simulink model "gm_DUALportRAMinterface_v3_vnl"  (R2024a)
settings: Solver=FixedStepDiscrete  StartTime=0.0  StopTime=20  RelTol=1e-3
undefined symbols (not defined in the file or in its folder): magnitude, Ts
libraries: hdlsllib x419, hdlmdlgenlib x103, embmathops x12, simulink x5, dsphdlxfrm2 x2
(part 11 of 11)

== system gm_DUALportRAMinterface_v3_vnl/PL_vnl/integration_block1/GA_main/coefficent_array1/individual1/Subsystem6 ==
  reg_in : Inport
  enable : Inport  Port=2
  Delay : Delay  DelayLength=1  InitialCondition=0  SampleTime=Ts
  Switch : Switch  Criteria=u2 > Threshold  SaturateOnIntegerOverflow=off  InputSameDT=off
  reg_out : Outport
  wires:
  reg_in/1 -> Switch/1
  enable/1 -> Switch/2
  Switch/1 -> Delay/1
  Delay/1 -> Switch/3, reg_out/1

== system gm_DUALportRAMinterface_v3_vnl/PL_vnl/integration_block1/GA_main/coefficent_array1/individual2/Subsystem ==
  reg_in : Inport
  enable : Inport  Port=2
  Delay : Delay  DelayLength=1  InitialCondition=0  SampleTime=Ts
  Switch : Switch  Criteria=u2 > Threshold  SaturateOnIntegerOverflow=off  InputSameDT=off
  reg_out : Outport
  wires:
  reg_in/1 -> Switch/1
  enable/1 -> Switch/2
  Switch/1 -> Delay/1
  Delay/1 -> Switch/3, reg_out/1

== system gm_DUALportRAMinterface_v3_vnl/PL_vnl/integration_block1/GA_main/coefficent_array1/individual2/Subsystem1 ==
  reg_in : Inport
  enable : Inport  Port=2
  Delay : Delay  DelayLength=1  InitialCondition=0  SampleTime=Ts
  Switch : Switch  Criteria=u2 > Threshold  SaturateOnIntegerOverflow=off  InputSameDT=off
  reg_out : Outport
  wires:
  reg_in/1 -> Switch/1
  enable/1 -> Switch/2
  Switch/1 -> Delay/1
  Delay/1 -> Switch/3, reg_out/1

== system gm_DUALportRAMinterface_v3_vnl/PL_vnl/integration_block1/GA_main/coefficent_array1/individual2/Subsystem2 ==
  reg_in : Inport
  enable : Inport  Port=2
  Delay : Delay  DelayLength=1  InitialCondition=0  SampleTime=Ts
  Switch : Switch  Criteria=u2 > Threshold  SaturateOnIntegerOverflow=off  InputSameDT=off
  reg_out : Outport
  wires:
  reg_in/1 -> Switch/1
  enable/1 -> Switch/2
  Switch/1 -> Delay/1
  Delay/1 -> Switch/3, reg_out/1

== system gm_DUALportRAMinterface_v3_vnl/PL_vnl/integration_block1/GA_main/coefficent_array1/individual2/Subsystem3 ==
  reg_in : Inport
  enable : Inport  Port=2
  Delay : Delay  DelayLength=1  InitialCondition=0  SampleTime=Ts
  Switch : Switch  Criteria=u2 > Threshold  SaturateOnIntegerOverflow=off  InputSameDT=off
  reg_out : Outport
  wires:
  reg_in/1 -> Switch/1
  enable/1 -> Switch/2
  Switch/1 -> Delay/1
  Delay/1 -> Switch/3, reg_out/1

== system gm_DUALportRAMinterface_v3_vnl/PL_vnl/integration_block1/GA_main/coefficent_array1/individual2/Subsystem4 ==
  reg_in : Inport
  enable : Inport  Port=2
  Delay : Delay  DelayLength=1  InitialCondition=0  SampleTime=Ts
  Switch : Switch  Criteria=u2 > Threshold  SaturateOnIntegerOverflow=off  InputSameDT=off
  reg_out : Outport
  wires:
  reg_in/1 -> Switch/1
  enable/1 -> Switch/2
  Switch/1 -> Delay/1
  Delay/1 -> Switch/3, reg_out/1

== system gm_DUALportRAMinterface_v3_vnl/PL_vnl/integration_block1/GA_main/coefficent_array1/individual2/Subsystem5 ==
  reg_in : Inport
  enable : Inport  Port=2
  Delay : Delay  DelayLength=1  InitialCondition=0  SampleTime=Ts
  Switch : Switch  Criteria=u2 > Threshold  SaturateOnIntegerOverflow=off  InputSameDT=off
  reg_out : Outport
  wires:
  reg_in/1 -> Switch/1
  enable/1 -> Switch/2
  Switch/1 -> Delay/1
  Delay/1 -> Switch/3, reg_out/1

== system gm_DUALportRAMinterface_v3_vnl/PL_vnl/integration_block1/GA_main/coefficent_array1/individual2/Subsystem6 ==
  reg_in : Inport
  enable : Inport  Port=2
  Delay : Delay  DelayLength=1  InitialCondition=0  SampleTime=Ts
  Switch : Switch  Criteria=u2 > Threshold  SaturateOnIntegerOverflow=off  InputSameDT=off
  reg_out : Outport
  wires:
  Delay/1 -> reg_out/1, Switch/3
  Switch/1 -> Delay/1
  enable/1 -> Switch/2
  reg_in/1 -> Switch/1

== system gm_DUALportRAMinterface_v3_vnl/PL_vnl/integration_block1/GA_main/coefficent_array1/individual3/Subsystem ==
  reg_in : Inport
  enable : Inport  Port=2
  Delay : Delay  DelayLength=1  InitialCondition=0  SampleTime=Ts
  Switch : Switch  Criteria=u2 > Threshold  SaturateOnIntegerOverflow=off  InputSameDT=off
  reg_out : Outport
  wires:
  Delay/1 -> reg_out/1, Switch/3
  Switch/1 -> Delay/1
  enable/1 -> Switch/2
  reg_in/1 -> Switch/1

== system gm_DUALportRAMinterface_v3_vnl/PL_vnl/integration_block1/GA_main/coefficent_array1/individual3/Subsystem1 ==
  reg_in : Inport
  enable : Inport  Port=2
  Delay : Delay  DelayLength=1  InitialCondition=0  SampleTime=Ts
  Switch : Switch  Criteria=u2 > Threshold  SaturateOnIntegerOverflow=off  InputSameDT=off
  reg_out : Outport
  wires:
  Delay/1 -> reg_out/1, Switch/3
  Switch/1 -> Delay/1
  enable/1 -> Switch/2
  reg_in/1 -> Switch/1

== system gm_DUALportRAMinterface_v3_vnl/PL_vnl/integration_block1/GA_main/coefficent_array1/individual3/Subsystem2 ==
  reg_in : Inport
  enable : Inport  Port=2
  Delay : Delay  DelayLength=1  InitialCondition=0  SampleTime=Ts
  Switch : Switch  Criteria=u2 > Threshold  SaturateOnIntegerOverflow=off  InputSameDT=off
  reg_out : Outport
  wires:
  Delay/1 -> reg_out/1, Switch/3
  Switch/1 -> Delay/1
  enable/1 -> Switch/2
  reg_in/1 -> Switch/1

== system gm_DUALportRAMinterface_v3_vnl/PL_vnl/integration_block1/GA_main/coefficent_array1/individual3/Subsystem3 ==
  reg_in : Inport
  enable : Inport  Port=2
  Delay : Delay  DelayLength=1  InitialCondition=0  SampleTime=Ts
  Switch : Switch  Criteria=u2 > Threshold  SaturateOnIntegerOverflow=off  InputSameDT=off
  reg_out : Outport
  wires:
  Delay/1 -> reg_out/1, Switch/3
  Switch/1 -> Delay/1
  enable/1 -> Switch/2
  reg_in/1 -> Switch/1

== system gm_DUALportRAMinterface_v3_vnl/PL_vnl/integration_block1/GA_main/coefficent_array1/individual3/Subsystem4 ==
  reg_in : Inport
  enable : Inport  Port=2
  Delay : Delay  DelayLength=1  InitialCondition=0  SampleTime=Ts
  Switch : Switch  Criteria=u2 > Threshold  SaturateOnIntegerOverflow=off  InputSameDT=off
  reg_out : Outport
  wires:
  Delay/1 -> reg_out/1, Switch/3
  Switch/1 -> Delay/1
  enable/1 -> Switch/2
  reg_in/1 -> Switch/1

== system gm_DUALportRAMinterface_v3_vnl/PL_vnl/integration_block1/GA_main/coefficent_array1/individual3/Subsystem5 ==
  reg_in : Inport
  enable : Inport  Port=2
  Delay : Delay  DelayLength=1  InitialCondition=0  SampleTime=Ts
  Switch : Switch  Criteria=u2 > Threshold  SaturateOnIntegerOverflow=off  InputSameDT=off
  reg_out : Outport
  wires:
  Delay/1 -> reg_out/1, Switch/3
  Switch/1 -> Delay/1
  enable/1 -> Switch/2
  reg_in/1 -> Switch/1

== system gm_DUALportRAMinterface_v3_vnl/PL_vnl/integration_block1/GA_main/coefficent_array1/individual3/Subsystem6 ==
  reg_in : Inport
  enable : Inport  Port=2
  Delay : Delay  DelayLength=1  InitialCondition=0  SampleTime=Ts
  Switch : Switch  Criteria=u2 > Threshold  SaturateOnIntegerOverflow=off  InputSameDT=off
  reg_out : Outport
  wires:
  reg_in/1 -> Switch/1
  enable/1 -> Switch/2
  Switch/1 -> Delay/1
  Delay/1 -> Switch/3, reg_out/1

== system gm_DUALportRAMinterface_v3_vnl/PL_vnl/integration_block1/GA_main/coefficent_array1/individual4/Subsystem ==
  reg_in : Inport
  enable : Inport  Port=2
  Delay : Delay  DelayLength=1  InitialCondition=0  SampleTime=Ts
  Switch : Switch  Criteria=u2 > Threshold  SaturateOnIntegerOverflow=off  InputSameDT=off
  reg_out : Outport
  wires:
  reg_in/1 -> Switch/1
  enable/1 -> Switch/2
  Switch/1 -> Delay/1
  Delay/1 -> Switch/3, reg_out/1

== system gm_DUALportRAMinterface_v3_vnl/PL_vnl/integration_block1/GA_main/coefficent_array1/individual4/Subsystem1 ==
  reg_in : Inport
  enable : Inport  Port=2
  Delay : Delay  DelayLength=1  InitialCondition=0  SampleTime=Ts
  Switch : Switch  Criteria=u2 > Threshold  SaturateOnIntegerOverflow=off  InputSameDT=off
  reg_out : Outport
  wires:
  reg_in/1 -> Switch/1
  enable/1 -> Switch/2
  Switch/1 -> Delay/1
  Delay/1 -> Switch/3, reg_out/1

== system gm_DUALportRAMinterface_v3_vnl/PL_vnl/integration_block1/GA_main/coefficent_array1/individual4/Subsystem2 ==
  reg_in : Inport
  enable : Inport  Port=2
  Delay : Delay  DelayLength=1  InitialCondition=0  SampleTime=Ts
  Switch : Switch  Criteria=u2 > Threshold  SaturateOnIntegerOverflow=off  InputSameDT=off
  reg_out : Outport
  wires:
  reg_in/1 -> Switch/1
  enable/1 -> Switch/2
  Switch/1 -> Delay/1
  Delay/1 -> Switch/3, reg_out/1

== system gm_DUALportRAMinterface_v3_vnl/PL_vnl/integration_block1/GA_main/coefficent_array1/individual4/Subsystem3 ==
  reg_in : Inport
  enable : Inport  Port=2
  Delay : Delay  DelayLength=1  InitialCondition=0  SampleTime=Ts
  Switch : Switch  Criteria=u2 > Threshold  SaturateOnIntegerOverflow=off  InputSameDT=off
  reg_out : Outport
  wires:
  reg_in/1 -> Switch/1
  enable/1 -> Switch/2
  Switch/1 -> Delay/1
  Delay/1 -> Switch/3, reg_out/1

== system gm_DUALportRAMinterface_v3_vnl/PL_vnl/integration_block1/GA_main/coefficent_array1/individual4/Subsystem4 ==
  reg_in : Inport
  enable : Inport  Port=2
  Delay : Delay  DelayLength=1  InitialCondition=0  SampleTime=Ts
  Switch : Switch  Criteria=u2 > Threshold  SaturateOnIntegerOverflow=off  InputSameDT=off
  reg_out : Outport
  wires:
  reg_in/1 -> Switch/1
  enable/1 -> Switch/2
  Switch/1 -> Delay/1
  Delay/1 -> Switch/3, reg_out/1

== system gm_DUALportRAMinterface_v3_vnl/PL_vnl/integration_block1/GA_main/coefficent_array1/individual4/Subsystem5 ==
  reg_in : Inport
  enable : Inport  Port=2
  Delay : Delay  DelayLength=1  InitialCondition=0  SampleTime=Ts
  Switch : Switch  Criteria=u2 > Threshold  SaturateOnIntegerOverflow=off  InputSameDT=off
  reg_out : Outport
  wires:
  reg_in/1 -> Switch/1
  enable/1 -> Switch/2
  Switch/1 -> Delay/1
  Delay/1 -> Switch/3, reg_out/1

== system gm_DUALportRAMinterface_v3_vnl/PL_vnl/integration_block1/GA_main/coefficent_array1/individual4/Subsystem6 ==
  reg_in : Inport
  enable : Inport  Port=2
  Delay : Delay  DelayLength=1  InitialCondition=0  SampleTime=Ts
  Switch : Switch  Criteria=u2 > Threshold  SaturateOnIntegerOverflow=off  InputSameDT=off
  reg_out : Outport
  wires:
  Delay/1 -> reg_out/1, Switch/3
  Switch/1 -> Delay/1
  enable/1 -> Switch/2
  reg_in/1 -> Switch/1

== stateflow chart gm_DUALportRAMinterface_v3_vnl/PL/integration_block1/FIFO_system3/Chart1/Chart1 ==
  settings: updateMethod=DISCRETE  sampleTime=Ts  executeAtInitialization=1
  state initial_counter
    during:
    enable_counter = false;
  state counter_state
    during:
    enable_counter = true;
  (default) -> initial_counter
  counter_state -> initial_counter : [counter == 1+(4096+2048+1)]
  initial_counter -> counter_state : [en_out == true]
  data: counter input fixdt(0,13,0); enable_counter output boolean; en_out input boolean

== stateflow chart gm_DUALportRAMinterface_v3_vnl/PL/integration_block1/FIFO_system3/Chart2/Chart2 ==
  settings: updateMethod=DISCRETE  sampleTime=Ts  executeAtInitialization=1
  state initial_push
    during:
    enable_push = false;
  state push_state
    during:
    enable_push = true;
  (default) -> initial_push
  push_state -> initial_push : [full == true]
  initial_push -> push_state : [load_FIFO1 == true]
  data: load_FIFO1 input boolean; full input boolean; enable_push output boolean

== stateflow chart gm_DUALportRAMinterface_v3_vnl/PL/integration_block1/FIFO_system1/Chart3/Chart3 ==
  settings: updateMethod=DISCRETE  sampleTime=Ts  executeAtInitialization=1
  state initial_popstate
    during:
    enable_pop = false;
  state pop_state
    during:
    enable_pop = true;
  (default) -> initial_popstate
  pop_state -> initial_popstate : [counter == 2+(4096+2048+1)]
  initial_popstate -> pop_state : [counter == 1]
  data: enable_pop output boolean; counter input fixdt(0,13,0)

== stateflow chart gm_DUALportRAMinterface_v3_vnl/PL/integration_block1/FIFO_system3/Chart3/Chart3 ==
  settings: updateMethod=DISCRETE  sampleTime=Ts  executeAtInitialization=1
  state initial_popstate
    during:
    enable_pop = false;
  state pop_state
    during:
    enable_pop = true;
  (default) -> initial_popstate
  pop_state -> initial_popstate : [counter == 2+(4096+2048+1)]
  initial_popstate -> pop_state : [counter == 1]
  data: enable_pop output boolean; counter input fixdt(0,13,0)

== stateflow chart gm_DUALportRAMinterface_v3_vnl/PL/integration_block1/FIFO_system1/Chart1/Chart1 ==
  settings: updateMethod=DISCRETE  sampleTime=Ts  executeAtInitialization=1
  state initial_counter
    during:
    enable_counter = false;
  state counter_state
    during:
    enable_counter = true;
  (default) -> initial_counter
  counter_state -> initial_counter : [counter == 1+(4096+2048+1)]
  initial_counter -> counter_state : [en_out == true]
  data: counter input fixdt(0,13,0); enable_counter output boolean; en_out input boolean

== stateflow chart gm_DUALportRAMinterface_v3_vnl/PL/integration_block1/FIFO_system1/Chart2/Chart2 ==
  settings: updateMethod=DISCRETE  sampleTime=Ts  executeAtInitialization=1
  state initial_push
    during:
    enable_push = false;
  state push_state
    during:
    enable_push = true;
  (default) -> initial_push
  push_state -> initial_push : [full == true]
  initial_push -> push_state : [load_FIFO1 == true]
  data: load_FIFO1 input boolean; full input boolean; enable_push output boolean

== stateflow chart gm_DUALportRAMinterface_v3_vnl/PL/Chart/Chart ==
  settings: executeAtInitialization=1
  state initial_wait_state
    entry:
    counter_increment = false;
    counter_reset = true;
    write_enable = false;
  state PL_read_data
    entry:
    counter_increment = true;
    counter_reset = false;
    write_enable = false;
  state wait_for_GA_done
    entry:
    counter_increment = false;
    counter_reset = true;
    write_enable = false;
  state reset_state
    entry:
    counter_increment = false;
    counter_reset = true;
    write_enable = false;
  state PL_write_data_back
    entry:
    counter_increment = true;
    counter_reset = false;
    write_enable = true;
  (default) -> initial_wait_state
  initial_wait_state -> PL_read_data : [GPIO == 1]
  reset_state -> initial_wait_state
  PL_read_data -> wait_for_GA_done : [counter == (4096+2048+1)*2]
  wait_for_GA_done -> PL_write_data_back : [GA_done == 1]
  PL_write_data_back -> reset_state : [counter == 8]
  data: GA_done input boolean; GPIO input; counter input; counter_increment output boolean; counter_reset output boolean; write_enable output boolean

== stateflow chart gm_DUALportRAMinterface_v3_vnl/PL_vnl/Chart ==
  settings: executeAtInitialization=1
  state initial_wait_state
    entry:
    counter_increment = false;
    counter_reset = true;
    write_enable = false;
  state PL_read_data
    entry:
    counter_increment = true;
    counter_reset = false;
    write_enable = false;
  state wait_for_GA_done
    entry:
    counter_increment = false;
    counter_reset = true;
    write_enable = false;
  state reset_state
    entry:
    counter_increment = false;
    counter_reset = true;
    write_enable = false;
  state PL_write_data_back
    entry:
    counter_increment = true;
    counter_reset = false;
    write_enable = true;
  (default) -> initial_wait_state
  initial_wait_state -> PL_read_data : [GPIO == 1]
  reset_state -> initial_wait_state
  PL_read_data -> wait_for_GA_done : [counter == (4096+2048+1)*2]
  wait_for_GA_done -> PL_write_data_back : [GA_done == 1]
  PL_write_data_back -> reset_state : [counter == 8]
  data: GA_done input boolean; GPIO input; counter input; counter_increment output boolean; counter_reset output boolean; write_enable output boolean

== stateflow chart gm_DUALportRAMinterface_v3_vnl/PL_vnl/integration_block1/FIFO_system1/Chart1 ==
  settings: updateMethod=DISCRETE  sampleTime=Ts  executeAtInitialization=1
  state initial_counter
    during:
    enable_counter = false;
  state counter_state
    during:
    enable_counter = true;
  (default) -> initial_counter
  counter_state -> initial_counter : [counter == 1+(4096+2048+1)]
  initial_counter -> counter_state : [en_out == true]
  data: counter input fixdt(0,13,0); enable_counter output boolean; en_out input boolean

== stateflow chart gm_DUALportRAMinterface_v3_vnl/PL_vnl/integration_block1/FIFO_system1/Chart2 ==
  settings: updateMethod=DISCRETE  sampleTime=Ts  executeAtInitialization=1
  state initial_push
    during:
    enable_push = false;
  state push_state
    during:
    enable_push = true;
  (default) -> initial_push
  push_state -> initial_push : [full == true]
  initial_push -> push_state : [load_FIFO1 == true]
  data: load_FIFO1 input boolean; full input boolean; enable_push output boolean

== stateflow chart gm_DUALportRAMinterface_v3_vnl/PL_vnl/integration_block1/FIFO_system1/Chart3 ==
  settings: updateMethod=DISCRETE  sampleTime=Ts  executeAtInitialization=1
  state initial_popstate
    during:
    enable_pop = false;
  state pop_state
    during:
    enable_pop = true;
  (default) -> initial_popstate
  pop_state -> initial_popstate : [counter == 2+(4096+2048+1)]
  initial_popstate -> pop_state : [counter == 1]
  data: enable_pop output boolean; counter input fixdt(0,13,0)

== stateflow chart gm_DUALportRAMinterface_v3_vnl/PL_vnl/integration_block1/FIFO_system3/Chart1 ==
  settings: updateMethod=DISCRETE  sampleTime=Ts  executeAtInitialization=1
  state initial_counter
    during:
    enable_counter = false;
  state counter_state
    during:
    enable_counter = true;
  (default) -> initial_counter
  counter_state -> initial_counter : [counter == 1+(4096+2048+1)]
  initial_counter -> counter_state : [en_out == true]
  data: counter input fixdt(0,13,0); enable_counter output boolean; en_out input boolean

== stateflow chart gm_DUALportRAMinterface_v3_vnl/PL_vnl/integration_block1/FIFO_system3/Chart2 ==
  settings: updateMethod=DISCRETE  sampleTime=Ts  executeAtInitialization=1
  state initial_push
    during:
    enable_push = false;
  state push_state
    during:
    enable_push = true;
  (default) -> initial_push
  push_state -> initial_push : [full == true]
  initial_push -> push_state : [load_FIFO1 == true]
  data: load_FIFO1 input boolean; full input boolean; enable_push output boolean

== stateflow chart gm_DUALportRAMinterface_v3_vnl/PL/integration_block1/GA_main/Chart/Chart ==
  settings: executeAtInitialization=1
  state index_and_hold
    entry:
    index_increment = true;
    slave_input = false;
    master_input = false;
    FIFO_out_en = false;
    exit:
    index_increment = false;
  state Enable_load_fifo
    load_fifo = true;
  state wait_for_FIFO
    load_fifo = false;
  state score_population
    entry:
    GA_done = false;
    a2_method = 1;
    a3_method = 1;
    a4_method = 1;
    b2_method = 1;
    b3_method = 1;
    b4_method = 1;
    slave_input = false;
    slave_output = true;
    master_input = true;
    master_output = 0;
    master_sort = false;
    generation_increment = false;
    generation_reset = false;
    index_increment = false;
    index_reset = false;
    FIFO_out_en = true;
  state initial_state
    during:
    GA_done = false;
    a2_method = 1;
    a3_method = 1;
    a4_method = 1;
    b2_method = 1;
    b3_method = 1;
    b4_method = 1;
    slave_input = false;
    slave_output = false;
    master_input = false;
    master_output = 0;
    master_sort = false;
    generation_increment = false;
    generation_reset = true;
    index_increment = false;
    index_reset = true;
    load_fifo = false;
    FIFO_out_en = false;
  state initial_random_population
    during:
    GA_done = false;
    a2_method = 1;
    a3_method = 1;
    a4_method = 1;
    b2_method = 1;
    b3_method = 1;
    b4_method = 1;
    slave_input = true;
    slave_output = false;
    master_input = false;
    master_output = 0;
    master_sort = false;
    generation_increment = false;
    generation_reset = false;
    index_increment = true;
    index_reset = false;
  state start_index_and_hold
    entry:
    index_reset = true;
    index_increment = true;
    slave_input = false;
    generation_increment = false;
    exit:
    index_increment = false;
    index_reset = false;
  state New_individual
    entry:
    a2_method = 1;
    a3_method = 1;
    a4_method = 1;
    b2_method = 1;
    b3_method = 1;
    b4_method = 1;
    slave_input = true;
    slave_output = false;
    master_input = false;
    master_output = 1;
    master_sort = false;
    generation_increment = false;
    generation_reset = false;
    index_increment = false;
    index_reset = false;
  state sort_population
    entry:
    slave_input = false;
    slave_output = false;
    master_input = false;
    master_output = 0;
    master_sort = true;
    generation_increment = false;
    generation_reset = false;
    index_increment = false;
    index_reset = true;
    FIFO_out_en = false;
  state Eliteism_or_Replication
    entry:
    a2_method = 3;
    a3_method = 3;
    a4_method = 3;
    b2_method = 3;
    b3_method = 3;
    b4_method = 3;
    slave_input = true;
    slave_output = false;
    master_input = false;
    master_output = 1;
    master_sort = false;
    generation_increment = false;
    generation_reset = false;
    index_increment = false;
    index_reset = false;
  state generation_update
    entry:
    slave_input = false;
    slave_output = false;
    master_input = false;
    master_output = 0;
    master_sort = false;
    generation_increment = true;
    generation_reset = false;
    index_increment = false;
    index_reset = true;
  state index_update
    entry:
    slave_input = false;
    slave_output = false;
    master_input = false;
    master_output = 0;
    master_sort = false;
    generation_increment = false;
    generation_reset = false;
    index_increment = true;
    index_reset = false;
  state GA_done_state
    entry:
    GA_done = true;
  state Crossover_load_dad
    entry:
    a2_method = 3;
    a3_method = 3;
    a4_method = 3;
    b2_method = 3;
    b3_method = 3;
    b4_method = 3;
    slave_input = false;
    slave_output = false;
    master_input = false;
    master_output = 2;
    master_sort = false;
    generation_increment = false;
    generation_reset = false;
    index_increment = false;
    index_reset = false;
  state Mutation1
    entry:
    a2_method = 1;
    a3_method = 3;
    a4_method = 3;
    b2_method = 3;
    b3_method = 3;
    b4_method = 3;
    slave_input = true;
    slave_output = false;
    master_input = false;
    master_output = 1;
    master_sort = false;
    generation_increment = false;
    generation_reset = false;
    index_increment = false;
    index_reset = false;
  state Mutation2
    entry:
    a2_method = 3;
    a3_method = 1;
    a4_method = 3;
    b2_method = 3;
    b3_method = 3;
    b4_method = 3;
    slave_input = true;
    slave_output = false;
    master_input = false;
    master_output = 1;
    master_sort = false;
    generation_increment = false;
    generation_reset = false;
    index_increment = false;
    index_reset = false;
  state Mutation3
    entry:
    a2_method = 3;
    a3_method = 3;
    a4_method = 1;
    b2_method = 3;
    b3_method = 3;
    b4_method = 3;
    slave_input = true;
    slave_output = false;
    master_input = false;
    master_output = 1;
    master_sort = false;
    generation_increment = false;
    generation_reset = false;
    index_increment = false;
    index_reset = false;
  state Mutation4
    entry:
    a2_method = 3;
    a3_method = 3;
    a4_method = 3;
    b2_method = 1;
    b3_method = 3;
    b4_method = 3;
    slave_input = true;
    slave_output = false;
    master_input = false;
    master_output = 1;
    master_sort = false;
    generation_increment = false;
    generation_reset = false;
    index_increment = false;
    index_reset = false;
  state Mutation5
    entry:
    a2_method = 3;
    a3_method = 3;
    a4_method = 3;
    b2_method = 3;
    b3_method = 1;
    b4_method = 3;
    slave_input = true;
    slave_output = false;
    master_input = false;
    master_output = 1;
    master_sort = false;
    generation_increment = false;
    generation_reset = false;
    index_increment = false;
    index_reset = false;
  state Mutation6
    entry:
    a2_method = 3;
    a3_method = 3;
    a4_method = 3;
    b2_method = 3;
    b3_method = 3;
    b4_method = 1;
    slave_input = true;
    slave_output = false;
    master_input = false;
    master_output = 1;
    master_sort = false;
    generation_increment = false;
    generation_reset = false;
    index_increment = false;
    index_reset = false;
  state Crossover1
    entry:
    a2_method = 2;
    a3_method = 3;
    a4_method = 3;
    b2_method = 3;
    b3_method = 3;
    b4_method = 3;
    slave_input = true;
    slave_output = false;
    master_input = false;
    master_output = 1;
    master_sort = false;
    generation_increment = false;
    generation_reset = false;
    index_increment = false;
    index_reset = false;
  state Crossover2
    entry:
    a2_method = 2;
    a3_method = 2;
    a4_method = 3;
    b2_method = 3;
    b3_method = 3;
    b4_method = 3;
    slave_input = true;
    slave_output = false;
    master_input = false;
    master_output = 1;
    master_sort = false;
    generation_increment = false;
    generation_reset = false;
    index_increment = false;
    index_reset = false;
  state Crossover3
    entry:
    a2_method = 2;
    a3_method = 2;
    a4_method = 2;
    b2_method = 3;
    b3_method = 3;
    b4_method = 3;
    slave_input = true;
    slave_output = false;
    master_input = false;
    master_output = 1;
    master_sort = false;
    generation_increment = false;
    generation_reset = false;
    index_increment = false;
    index_reset = false;
  state Crossover4
    entry:
    a2_method = 2;
    a3_method = 2;
    a4_method = 2;
    b2_method = 2;
    b3_method = 3;
    b4_method = 3;
    slave_input = true;
    slave_output = false;
    master_input = false;
    master_output = 1;
    master_sort = false;
    generation_increment = false;
    generation_reset = false;
    index_increment = false;
    index_reset = false;
  state Crossover5
    entry:
    a2_method = 2;
    a3_method = 2;
    a4_method = 2;
    b2_method = 2;
    b3_method = 2;
    b4_method = 3;
    slave_input = true;
    slave_output = false;
    master_input = false;
    master_output = 1;
    master_sort = false;
    generation_increment = false;
    generation_reset = false;
    index_increment = false;
    index_reset = false;
  Enable_load_fifo -> wait_for_FIFO
  score_population -> index_and_hold [order 2] : [score_done == 1]
  index_and_hold -> score_population
  (default) -> initial_state [order 1]
  initial_state -> Enable_load_fifo : [start_GA==1]
  wait_for_FIFO -> initial_random_population : [FIFO_full == 1]
  initial_random_population -> start_index_and_hold : [sample_index == 5]
  start_index_and_hold -> score_population
  generation_update -> start_index_and_hold [order 2]
  score_population -> sort_population [order 1] : [sample_index==4 & score_done==1]
  New_individual -> (junction 296)
  GA_done_state -> initial_state
  (junction 296) -> (junction 297)
  (junction 289) -> New_individual
  (junction 287) -> (junction 289) : [selected_method==4]
  sort_population -> index_update : [sort_done==1]
  (junction 297) -> index_update
  index_update -> (junction 287) [order 4]
  Eliteism_or_Replication -> index_update
  index_update -> Eliteism_or_Replication [order 2] : [sample_index==1 | selected_method==1]
  generation_update -> GA_done_state [order 1] : [generation_counter==5000]
  index_update -> generation_update [order 1] : [sample_index==5]
  (junction 221) -> index_update
  (junction 227) -> (junction 221)
  (junction 229) -> (junction 227)
  (junction 231) -> (junction 229)
  (junction 272) -> (junction 231)
  Mutation2 -> (junction 221)
  Mutation3 -> (junction 227)
  Mutation4 -> (junction 229)
  Mutation5 -> (junction 231)
  Mutation6 -> (junction 272)
  (junction 236) -> index_update
  Mutation1 -> index_update
  index_update -> (junction 175) [order 3] : [selected_method==2]
  (default) -> Crossover_load_dad [order 2] : [selected_method==3]
  (junction 175) -> (junction 177) [order 1]
  (junction 177) -> (junction 178) [order 1]
  (junction 178) -> (junction 179) [order 1]
  (junction 179) -> (junction 180) [order 1]
  (junction 180) -> (junction 267) [order 2]
  (junction 175) -> Mutation1 [order 2] : [random_gene==1]
  (junction 177) -> Mutation2 [order 2] : [random_gene==2]
  (junction 178) -> Mutation3 [order 2] : [random_gene==3]
  (junction 179) -> Mutation4 [order 2] : [random_gene==4]
  (junction 180) -> Mutation5 [order 1] : [random_gene==5]
  (junction 267) -> Mutation6 : [random_gene==6]
  Crossover_load_dad -> (junction 212)
  (junction 237) -> (junction 236)
  (junction 239) -> (junction 237)
  (junction 241) -> (junction 239)
  (junction 277) -> (junction 241)
  Crossover1 -> (junction 236)
  Crossover2 -> (junction 237)
  Crossover3 -> (junction 239)
  Crossover4 -> (junction 241)
  Crossover5 -> (junction 277)
  (junction 212) -> (junction 213) [order 1]
  (junction 213) -> (junction 203) [order 1]
  (junction 203) -> (junction 210) [order 1]
  (junction 210) -> (junction 271) [order 2]
  (junction 212) -> Crossover1 [order 2] : [random_gene==1]
  (junction 213) -> Crossover2 [order 2] : [random_gene==2]
  (junction 203) -> Crossover3 [order 2] : [random_gene==3]
  (junction 210) -> Crossover4 [order 1] : [random_gene==4]
  (junction 271) -> Crossover5 : [random_gene==5|random_gene==6]
  data: GA_done output boolean; index_reset output boolean; index_increment output boolean; a2_method output fixdt(0,2,0); a3_method output fixdt(0,2,0); a4_method output fixdt(0,2,0); b4_method output fixdt(0,2,0); b2_method output fixdt(0,2,0); b3_method output fixdt(0,2,0); sort_done input boolean; start_GA input boolean; score_done input boolean; FIFO_full input boolean; random_gene input fixdt(0,3,0); selected_method input fixdt(0,3,0); slave_input output boolean; slave_output output boolean; master_input output boolean; generation_increment output boolean; generation_reset output boolean; master_output output fixdt(0,2,0); master_sort output boolean; sample_index input fixdt(0,4,0); generation_counter input fixdt(0,16,0); FIFO_out_en output boolean; load_fifo output boolean

== stateflow chart gm_DUALportRAMinterface_v3_vnl/PL/integration_block1/GA_main/coefficent_array/Chart/Chart ==
  settings: executeAtInitialization=1
  state initial_sort
    during:
    index_increment = false;
    index_reset = true;
    swaps_increment = false;
    reset_swaps = true;
    sort_done = false;
  state round_increment
    entry:
    index_reset = true;
    reset_swaps = true;
  state not_perform_swap
    entry:
    commit_swap = 0;
  state start_round
    entry:
    reset_swaps = false;
    index_reset = false;
  state index_increment
    entry:
    index_increment = true;
    exit:
    index_increment = false;
  state perform_swap
    entry:
    commit_swap = index;
    swaps_increment = true;
    exit:
    commit_swap = 0;
    swaps_increment = false;
  state done_state
    entry:
    sort_done = true;
  (default) -> initial_sort
  done_state -> initial_sort
  initial_sort -> start_round : [start_sort]
  perform_swap -> round_increment [order 1] : [index == 3]
  not_perform_swap -> round_increment [order 3] : [index == 3]
  round_increment -> start_round
  start_round -> round_increment [order 2] : [index == 4]
  start_round -> not_perform_swap [order 1] : [swap_signal == false]
  not_perform_swap -> index_increment [order 1] : [index<3]
  not_perform_swap -> done_state [order 2] : [swaps_in == 0]
  start_round -> perform_swap [order 3] : [swap_signal == true]
  index_increment -> start_round
  perform_swap -> index_increment [order 2] : [index<3]
  data: index input; start_sort input; swaps_in input; index_increment output boolean; index_reset output boolean; sort_done output boolean; swap_signal input boolean; commit_swap output fixdt(0,4,0); swaps_increment output boolean; reset_swaps output boolean

== stateflow chart gm_DUALportRAMinterface_v3_vnl/PL/integration_block1/GA_main/coefficent_array1/Chart/Chart ==
  settings: executeAtInitialization=1
  state initial_sort
    during:
    index_increment = false;
    index_reset = true;
    swaps_increment = false;
    reset_swaps = true;
    sort_done = false;
  state round_increment
    entry:
    index_reset = true;
    reset_swaps = true;
  state not_perform_swap
    entry:
    commit_swap = 0;
  state start_round
    entry:
    reset_swaps = false;
    index_reset = false;
  state index_increment
    entry:
    index_increment = true;
    exit:
    index_increment = false;
  state perform_swap
    entry:
    commit_swap = index;
    swaps_increment = true;
    exit:
    commit_swap = 0;
    swaps_increment = false;
  state done_state
    entry:
    sort_done = true;
  (default) -> initial_sort
  done_state -> initial_sort
  initial_sort -> start_round : [start_sort]
  perform_swap -> round_increment [order 1] : [index == 3]
  not_perform_swap -> round_increment [order 3] : [index == 3]
  round_increment -> start_round
  start_round -> round_increment [order 2] : [index == 4]
  start_round -> not_perform_swap [order 1] : [swap_signal == false]
  not_perform_swap -> index_increment [order 1] : [index<3]
  not_perform_swap -> done_state [order 2] : [swaps_in == 0]
  start_round -> perform_swap [order 3] : [swap_signal == true]
  index_increment -> start_round
  perform_swap -> index_increment [order 2] : [index<3]
  data: index input; start_sort input; swaps_in input; index_increment output boolean; index_reset output boolean; sort_done output boolean; swap_signal input boolean; commit_swap output fixdt(0,4,0); swaps_increment output boolean; reset_swaps output boolean

== stateflow chart gm_DUALportRAMinterface_v3_vnl/PL_vnl/integration_block1/FIFO_system3/Chart3 ==
  settings: updateMethod=DISCRETE  sampleTime=Ts  executeAtInitialization=1
  state initial_popstate
    during:
    enable_pop = false;
  state pop_state
    during:
    enable_pop = true;
  (default) -> initial_popstate
  pop_state -> initial_popstate : [counter == 2+(4096+2048+1)]
  initial_popstate -> pop_state : [counter == 1]
  data: enable_pop output boolean; counter input fixdt(0,13,0)

== stateflow chart gm_DUALportRAMinterface_v3_vnl/PL_vnl/integration_block1/GA_main/Chart ==
  settings: executeAtInitialization=1
  state index_and_hold
    entry:
    index_increment = true;
    slave_input = false;
    master_input = false;
    FIFO_out_en = false;
    exit:
    index_increment = false;
  state Enable_load_fifo
    load_fifo = true;
  state wait_for_FIFO
    load_fifo = false;
  state score_population
    entry:
    GA_done = false;
    a2_method = 1;
    a3_method = 1;
    a4_method = 1;
    b2_method = 1;
    b3_method = 1;
    b4_method = 1;
    slave_input = false;
    slave_output = true;
    master_input = true;
    master_output = 0;
    master_sort = false;
    generation_increment = false;
    generation_reset = false;
    index_increment = false;
    index_reset = false;
    FIFO_out_en = true;
  state initial_state
    during:
    GA_done = false;
    a2_method = 1;
    a3_method = 1;
    a4_method = 1;
    b2_method = 1;
    b3_method = 1;
    b4_method = 1;
    slave_input = false;
    slave_output = false;
    master_input = false;
    master_output = 0;
    master_sort = false;
    generation_increment = false;
    generation_reset = true;
    index_increment = false;
    index_reset = true;
    load_fifo = false;
    FIFO_out_en = false;
  state initial_random_population
    during:
    GA_done = false;
    a2_method = 1;
    a3_method = 1;
    a4_method = 1;
    b2_method = 1;
    b3_method = 1;
    b4_method = 1;
    slave_input = true;
    slave_output = false;
    master_input = false;
    master_output = 0;
    master_sort = false;
    generation_increment = false;
    generation_reset = false;
    index_increment = true;
    index_reset = false;
  state start_index_and_hold
    entry:
    index_reset = true;
    index_increment = true;
    slave_input = false;
    generation_increment = false;
    exit:
    index_increment = false;
    index_reset = false;
  state New_individual
    entry:
    a2_method = 1;
    a3_method = 1;
    a4_method = 1;
    b2_method = 1;
    b3_method = 1;
    b4_method = 1;
    slave_input = true;
    slave_output = false;
    master_input = false;
    master_output = 1;
    master_sort = false;
    generation_increment = false;
    generation_reset = false;
    index_increment = false;
    index_reset = false;
  state sort_population
    entry:
    slave_input = false;
    slave_output = false;
    master_input = false;
    master_output = 0;
    master_sort = true;
    generation_increment = false;
    generation_reset = false;
    index_increment = false;
    index_reset = true;
    FIFO_out_en = false;
  state Eliteism_or_Replication
    entry:
    a2_method = 3;
    a3_method = 3;
    a4_method = 3;
    b2_method = 3;
    b3_method = 3;
    b4_method = 3;
    slave_input = true;
    slave_output = false;
    master_input = false;
    master_output = 1;
    master_sort = false;
    generation_increment = false;
    generation_reset = false;
    index_increment = false;
    index_reset = false;
  state generation_update
    entry:
    slave_input = false;
    slave_output = false;
    master_input = false;
    master_output = 0;
    master_sort = false;
    generation_increment = true;
    generation_reset = false;
    index_increment = false;
    index_reset = true;
  state index_update
    entry:
    slave_input = false;
    slave_output = false;
    master_input = false;
    master_output = 0;
    master_sort = false;
    generation_increment = false;
    generation_reset = false;
    index_increment = true;
    index_reset = false;
  state GA_done_state
    entry:
    GA_done = true;
  state Crossover_load_dad
    entry:
    a2_method = 3;
    a3_method = 3;
    a4_method = 3;
    b2_method = 3;
    b3_method = 3;
    b4_method = 3;
    slave_input = false;
    slave_output = false;
    master_input = false;
    master_output = 2;
    master_sort = false;
    generation_increment = false;
    generation_reset = false;
    index_increment = false;
    index_reset = false;
  state Mutation1
    entry:
    a2_method = 1;
    a3_method = 3;
    a4_method = 3;
    b2_method = 3;
    b3_method = 3;
    b4_method = 3;
    slave_input = true;
    slave_output = false;
    master_input = false;
    master_output = 1;
    master_sort = false;
    generation_increment = false;
    generation_reset = false;
    index_increment = false;
    index_reset = false;
  state Mutation2
    entry:
    a2_method = 3;
    a3_method = 1;
    a4_method = 3;
    b2_method = 3;
    b3_method = 3;
    b4_method = 3;
    slave_input = true;
    slave_output = false;
    master_input = false;
    master_output = 1;
    master_sort = false;
    generation_increment = false;
    generation_reset = false;
    index_increment = false;
    index_reset = false;
  state Mutation3
    entry:
    a2_method = 3;
    a3_method = 3;
    a4_method = 1;
    b2_method = 3;
    b3_method = 3;
    b4_method = 3;
    slave_input = true;
    slave_output = false;
    master_input = false;
    master_output = 1;
    master_sort = false;
    generation_increment = false;
    generation_reset = false;
    index_increment = false;
    index_reset = false;
  state Mutation4
    entry:
    a2_method = 3;
    a3_method = 3;
    a4_method = 3;
    b2_method = 1;
    b3_method = 3;
    b4_method = 3;
    slave_input = true;
    slave_output = false;
    master_input = false;
    master_output = 1;
    master_sort = false;
    generation_increment = false;
    generation_reset = false;
    index_increment = false;
    index_reset = false;
  state Mutation5
    entry:
    a2_method = 3;
    a3_method = 3;
    a4_method = 3;
    b2_method = 3;
    b3_method = 1;
    b4_method = 3;
    slave_input = true;
    slave_output = false;
    master_input = false;
    master_output = 1;
    master_sort = false;
    generation_increment = false;
    generation_reset = false;
    index_increment = false;
    index_reset = false;
  state Mutation6
    entry:
    a2_method = 3;
    a3_method = 3;
    a4_method = 3;
    b2_method = 3;
    b3_method = 3;
    b4_method = 1;
    slave_input = true;
    slave_output = false;
    master_input = false;
    master_output = 1;
    master_sort = false;
    generation_increment = false;
    generation_reset = false;
    index_increment = false;
    index_reset = false;
  state Crossover1
    entry:
    a2_method = 2;
    a3_method = 3;
    a4_method = 3;
    b2_method = 3;
    b3_method = 3;
    b4_method = 3;
    slave_input = true;
    slave_output = false;
    master_input = false;
    master_output = 1;
    master_sort = false;
    generation_increment = false;
    generation_reset = false;
    index_increment = false;
    index_reset = false;
  state Crossover2
    entry:
    a2_method = 2;
    a3_method = 2;
    a4_method = 3;
    b2_method = 3;
    b3_method = 3;
    b4_method = 3;
    slave_input = true;
    slave_output = false;
    master_input = false;
    master_output = 1;
    master_sort = false;
    generation_increment = false;
    generation_reset = false;
    index_increment = false;
    index_reset = false;
  state Crossover3
    entry:
    a2_method = 2;
    a3_method = 2;
    a4_method = 2;
    b2_method = 3;
    b3_method = 3;
    b4_method = 3;
    slave_input = true;
    slave_output = false;
    master_input = false;
    master_output = 1;
    master_sort = false;
    generation_increment = false;
    generation_reset = false;
    index_increment = false;
    index_reset = false;
  state Crossover4
    entry:
    a2_method = 2;
    a3_method = 2;
    a4_method = 2;
    b2_method = 2;
    b3_method = 3;
    b4_method = 3;
    slave_input = true;
    slave_output = false;
    master_input = false;
    master_output = 1;
    master_sort = false;
    generation_increment = false;
    generation_reset = false;
    index_increment = false;
    index_reset = false;
  state Crossover5
    entry:
    a2_method = 2;
    a3_method = 2;
    a4_method = 2;
    b2_method = 2;
    b3_method = 2;
    b4_method = 3;
    slave_input = true;
    slave_output = false;
    master_input = false;
    master_output = 1;
    master_sort = false;
    generation_increment = false;
    generation_reset = false;
    index_increment = false;
    index_reset = false;
  Enable_load_fifo -> wait_for_FIFO
  score_population -> index_and_hold [order 2] : [score_done == 1]
  index_and_hold -> score_population
  (default) -> initial_state [order 1]
  initial_state -> Enable_load_fifo : [start_GA==1]
  wait_for_FIFO -> initial_random_population : [FIFO_full == 1]
  initial_random_population -> start_index_and_hold : [sample_index == 5]
  start_index_and_hold -> score_population
  generation_update -> start_index_and_hold [order 2]
  score_population -> sort_population [order 1] : [sample_index==4 & score_done==1]
  New_individual -> (junction 296)
  GA_done_state -> initial_state
  (junction 296) -> (junction 297)
  (junction 289) -> New_individual
  (junction 287) -> (junction 289) : [selected_method==4]
  sort_population -> index_update : [sort_done==1]
  (junction 297) -> index_update
  index_update -> (junction 287) [order 4]
  Eliteism_or_Replication -> index_update
  index_update -> Eliteism_or_Replication [order 2] : [sample_index==1 | selected_method==1]
  generation_update -> GA_done_state [order 1] : [generation_counter==5000]
  index_update -> generation_update [order 1] : [sample_index==5]
  (junction 221) -> index_update
  (junction 227) -> (junction 221)
  (junction 229) -> (junction 227)
  (junction 231) -> (junction 229)
  (junction 272) -> (junction 231)
  Mutation2 -> (junction 221)
  Mutation3 -> (junction 227)
  Mutation4 -> (junction 229)
  Mutation5 -> (junction 231)
  Mutation6 -> (junction 272)
  (junction 236) -> index_update
  Mutation1 -> index_update
  index_update -> (junction 175) [order 3] : [selected_method==2]
  (default) -> Crossover_load_dad [order 2] : [selected_method==3]
  (junction 175) -> (junction 177) [order 1]
  (junction 177) -> (junction 178) [order 1]
  (junction 178) -> (junction 179) [order 1]
  (junction 179) -> (junction 180) [order 1]
  (junction 180) -> (junction 267) [order 2]
  (junction 175) -> Mutation1 [order 2] : [random_gene==1]
  (junction 177) -> Mutation2 [order 2] : [random_gene==2]
  (junction 178) -> Mutation3 [order 2] : [random_gene==3]
  (junction 179) -> Mutation4 [order 2] : [random_gene==4]
  (junction 180) -> Mutation5 [order 1] : [random_gene==5]
  (junction 267) -> Mutation6 : [random_gene==6]
  Crossover_load_dad -> (junction 212)
  (junction 237) -> (junction 236)
  (junction 239) -> (junction 237)
  (junction 241) -> (junction 239)
  (junction 277) -> (junction 241)
  Crossover1 -> (junction 236)
  Crossover2 -> (junction 237)
  Crossover3 -> (junction 239)
  Crossover4 -> (junction 241)
  Crossover5 -> (junction 277)
  (junction 212) -> (junction 213) [order 1]
  (junction 213) -> (junction 203) [order 1]
  (junction 203) -> (junction 210) [order 1]
  (junction 210) -> (junction 271) [order 2]
  (junction 212) -> Crossover1 [order 2] : [random_gene==1]
  (junction 213) -> Crossover2 [order 2] : [random_gene==2]
  (junction 203) -> Crossover3 [order 2] : [random_gene==3]
  (junction 210) -> Crossover4 [order 1] : [random_gene==4]
  (junction 271) -> Crossover5 : [random_gene==5|random_gene==6]
  data: GA_done output boolean; index_reset output boolean; index_increment output boolean; a2_method output fixdt(0,2,0); a3_method output fixdt(0,2,0); a4_method output fixdt(0,2,0); b4_method output fixdt(0,2,0); b2_method output fixdt(0,2,0); b3_method output fixdt(0,2,0); sort_done input boolean; start_GA input boolean; score_done input boolean; FIFO_full input boolean; random_gene input fixdt(0,3,0); selected_method input fixdt(0,3,0); slave_input output boolean; slave_output output boolean; master_input output boolean; generation_increment output boolean; generation_reset output boolean; master_output output fixdt(0,2,0); master_sort output boolean; sample_index input fixdt(0,4,0); generation_counter input fixdt(0,16,0); FIFO_out_en output boolean; load_fifo output boolean

== stateflow chart gm_DUALportRAMinterface_v3_vnl/PL_vnl/integration_block1/GA_main/coefficent_array/Chart ==
  settings: executeAtInitialization=1
  state initial_sort
    during:
    index_increment = false;
    index_reset = true;
    swaps_increment = false;
    reset_swaps = true;
    sort_done = false;
  state round_increment
    entry:
    index_reset = true;
    reset_swaps = true;
  state not_perform_swap
    entry:
    commit_swap = 0;
  state start_round
    entry:
    reset_swaps = false;
    index_reset = false;
  state index_increment
    entry:
    index_increment = true;
    exit:
    index_increment = false;
  state perform_swap
    entry:
    commit_swap = index;
    swaps_increment = true;
    exit:
    commit_swap = 0;
    swaps_increment = false;
  state done_state
    entry:
    sort_done = true;
  (default) -> initial_sort
  done_state -> initial_sort
  initial_sort -> start_round : [start_sort]
  perform_swap -> round_increment [order 1] : [index == 3]
  not_perform_swap -> round_increment [order 3] : [index == 3]
  round_increment -> start_round
  start_round -> round_increment [order 2] : [index == 4]
  start_round -> not_perform_swap [order 1] : [swap_signal == false]
  not_perform_swap -> index_increment [order 1] : [index<3]
  not_perform_swap -> done_state [order 2] : [swaps_in == 0]
  start_round -> perform_swap [order 3] : [swap_signal == true]
  index_increment -> start_round
  perform_swap -> index_increment [order 2] : [index<3]
  data: index input; start_sort input; swaps_in input; index_increment output boolean; index_reset output boolean; sort_done output boolean; swap_signal input boolean; commit_swap output fixdt(0,4,0); swaps_increment output boolean; reset_swaps output boolean

== stateflow chart gm_DUALportRAMinterface_v3_vnl/PL_vnl/integration_block1/GA_main/coefficent_array1/Chart ==
  settings: executeAtInitialization=1
  state initial_sort
    during:
    index_increment = false;
    index_reset = true;
    swaps_increment = false;
    reset_swaps = true;
    sort_done = false;
  state round_increment
    entry:
    index_reset = true;
    reset_swaps = true;
  state not_perform_swap
    entry:
    commit_swap = 0;
  state start_round
    entry:
    reset_swaps = false;
    index_reset = false;
  state index_increment
    entry:
    index_increment = true;
    exit:
    index_increment = false;
  state perform_swap
    entry:
    commit_swap = index;
    swaps_increment = true;
    exit:
    commit_swap = 0;
    swaps_increment = false;
  state done_state
    entry:
    sort_done = true;
  (default) -> initial_sort
  done_state -> initial_sort
  initial_sort -> start_round : [start_sort]
  perform_swap -> round_increment [order 1] : [index == 3]
  not_perform_swap -> round_increment [order 3] : [index == 3]
  round_increment -> start_round
  start_round -> round_increment [order 2] : [index == 4]
  start_round -> not_perform_swap [order 1] : [swap_signal == false]
  not_perform_swap -> index_increment [order 1] : [index<3]
  not_perform_swap -> done_state [order 2] : [swaps_in == 0]
  start_round -> perform_swap [order 3] : [swap_signal == true]
  index_increment -> start_round
  perform_swap -> index_increment [order 2] : [index<3]
  data: index input; start_sort input; swaps_in input; index_increment output boolean; index_reset output boolean; sort_done output boolean; swap_signal input boolean; commit_swap output fixdt(0,4,0); swaps_increment output boolean; reset_swaps output boolean
